simulink model "preliminary_Model"  (R2022b)
settings: Solver=FixedStepAuto  StartTime=0.0  StopTime=5  FixedStep=0.00001  RelTol=1e-3
model workspace (MAT data in the model file):
  g = 9.81
values from neighbouring files (symbols this model uses):
  A = [               0                ,        1        ,        0 ... (first row only)    [first_code.m]
  B = [ 0 ; -Km/(Ib+mw*l^2) ; Km*(Ib + Iw + mw*l^2)/(Iw*(Ib + mw*l^2)) ]    [first_code.m]
  C = [1 0 0; 0 1 0; 0 0 1]    [first_code.m]
  Cb = 1.02e-3    (= 0.00102)    [first_code.m]
  Cw = 0.05e-3    (= 5e-05)    [first_code.m]
  D = [0; 0; 0]    [first_code.m]
  Ib = 3.34e-3    (= 0.00334)    [first_code.m]
  Iw = 0.57e-3    (= 0.00057)    [first_code.m]
  l = 0.085    [first_code.m]
  lb = 0.075    [first_code.m]
  mb = 0.419    [first_code.m]
  mw = 0.204    [first_code.m]
libraries: slpidlib x3
settings Model: Creator=sAjaD  LastModifiedBy=Kian
settings SolverCC: AlgebraicLoopSolver=TrustRegion
settings DebuggingCC: UnconnectedInputMsg=warning  UnconnectedOutputMsg=warning  UnconnectedLineMsg=warning  SFMachineParentedDataDiag=warning  UnderSpecifiedDimensionMsg=warning
settings ModelReferenceCC: EnableRefExpFcnMdlSchedulingChecks=on

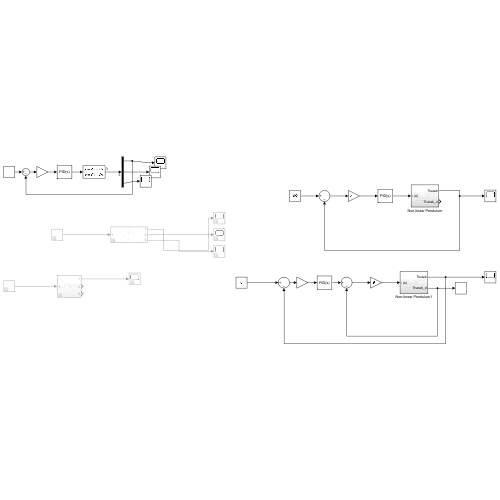
[thumbnail: Simulink's stored preview of the top-level diagram]
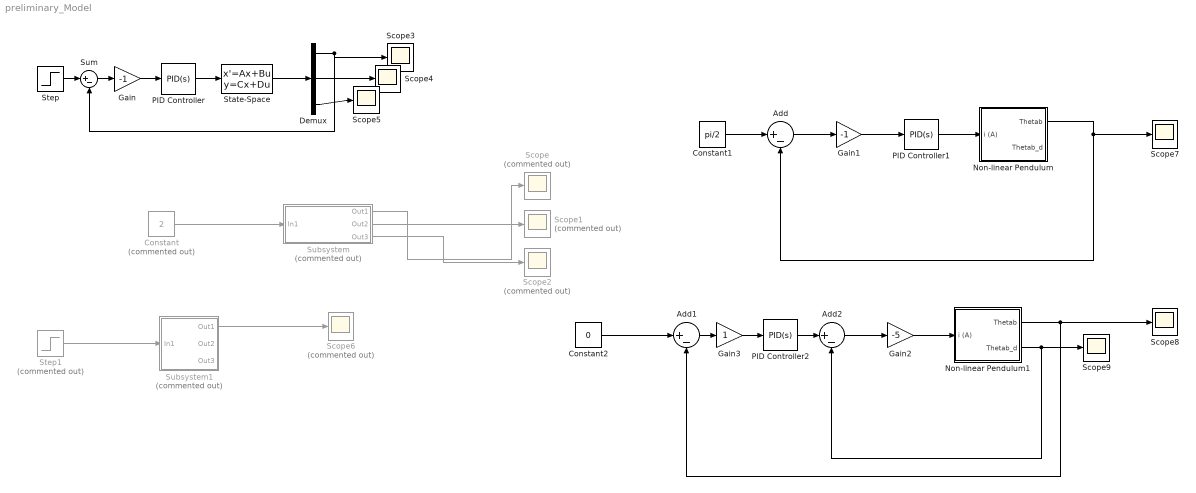
== system preliminary_Model ==
  Add : Sum  Inputs=|+-
  Add1 : Sum  Inputs=|+-
  Add2 : Sum  Inputs=|+-
  Constant : Constant  Commented=on  Value=2
  Constant1 : Constant  Value=pi/2
  Constant2 : Constant  Value=0
  Demux : Demux  Outputs=3
  Gain : Gain  Gain=-1
  Gain1 : Gain  Gain=-1
  Gain2 : Gain  Gain=-5
  Gain3 : Gain
  Non-linear Pendulum : Subsystem
  Non-linear Pendulum1 : Subsystem
  PID Controller : slpidlib/PID Controller  Controller=PID  Form=Parallel  TimeDomain=Continuous-time  UseExternalTs=off  SampleTime=-1  IntegratorMethod=Forward Euler  FilterMethod=Forward Euler  ControllerParametersSource=internal  P=100  I=0  UseKiTs=off  D=5  N=100  UseFilter=on  TunerSelectOption=Transfer Function Based (PID Tuner App)  InitialConditionSource=internal  InitialConditionForIntegrator=0  InitialConditionForFilter=0  DifferentiatorICPrevScaledInput=0  ExternalReset=none  TrackingMode=off  Kt=1  LimitOutput=off  SatLimitsSource=internal  UpperSaturationLimit=inf  LowerSaturationLimit=-inf  LinearizeAsGain=on  AntiWindupMode=none  Kb=1  LimitIntegrator=off  UpperIntegratorSaturationLimit=inf  LowerIntegratorSaturationLimit=-inf  POutMin=[]  POutMax=[]  IOutMin=[]  IOutMax=[]  DOutMin=[]  DOutMax=[]  NOutMin=[]  NOutMax=[]  SumOutMin=[]  SumOutMax=[]  SaturationOutMin=[]  SaturationOutMax=[]  PParamMin=[]  PParamMax=[]  IParamMin=[]  IParamMax=[]  DParamMin=[]  DParamMax=[]  NParamMin=[]  NParamMax=[]  KbParamMin=[]  KbParamMax=[]  KtParamMin=[]  KtParamMax=[]  KbOutMin=[]  KbOutMax=[]  KtOutMin=[]  KtOutMax=[]  IntegratorOutMin=[]  IntegratorOutMax=[]  FilterOutMin=[]  FilterOutMax=[]  SumI1OutMin=[]  SumI1OutMax=[]  SumI2OutMin=[]  SumI2OutMax=[]  SumI3OutMin=[]  SumI3OutMax=[]  SumI4OutMin=[]  SumI4OutMax=[]  SumDOutMin=[]  SumDOutMax=[]  DifferentiatorOutMin=[]  DifferentiatorOutMax=[]  FilterDiffOutCoefMin=[]  FilterDiffOutCoefMax=[]  ReciprocalOutMin=[]  ReciprocalOutMax=[]  SumDenOutMin=[]  SumDenOutMax=[]  SumNumOutMin=[]  SumNumOutMax=[]  DivideOutMin=[]  DivideOutMax=[]  UdiffTsProdOutMin=[]  UdiffTsProdOutMax=[]  NTsProdOutMin=[]  NTsProdOutMax=[]  UintegralTsProdOutMin=[]  UintegralTsProdOutMax=[]  UngainTsProdOutMin=[]  UngainTsProdOutMax=[]  ClampingZeroOutDataTypeStr=Inherit: Inherit via back propagation  ClampingZeroOutMin=[]  ClampingZeroOutMax=[]  FilterDenConstantOutDataTypeStr=Inherit: Inherit via back propagation  FilterDenConstantOutMin=[]  FilterDenConstantOutMax=[]  PCopyOutDataTypeStr=Inherit: Inherit via back propagation  PCopyOutMin=[]  PCopyOutMax=[]  NCopyOutDataTypeStr=Inherit: Inherit via back propagation  NCopyOutMin=[]  NCopyOutMax=[]  IntegratorContinuousStateAttributes=''  IntegratorStateMustResolveToSignalObject=off  IntegratorRTWStateStorageClass=Auto  FilterContinuousStateAttributes=''  FilterStateMustResolveToSignalObject=off  FilterRTWStateStorageClass=Auto  ParallelPVariant=InternalParameters  IdealPVariant=Disabled  IVariant=InternalParameters  DVariant=InternalParameters  IntegratorVariant=Continuous  SatVariant=Disabled  AWVariant=Passthrough  PCopyVariant=Disabled  TRVariant=Disabled  FdbkBlocksVariant=Forward  IdealPFdbkVariant=Disabled  SatFdbkVariant=Disabled  DerivativeFilterVariant=ContFilter  NVariant=InternalParameters  NCopyVariant=Disabled  FilterICVariant=InternalICsFilter  IntegratorICVariant=InternalICs  ExternalResetVariant=Disabled  TRSumVariant=Passthrough  SumFdbkVariant=Disabled  SumVariant=Sum_PID  TsampFilterVariant=InternalTs  TsampNgainVariant=Passthrough  TsampIntegralVariant=Passthrough  ExternalSaturationOutDataTypeStr=Inherit: Same as second input
  PID Controller1 : slpidlib/PID Controller  Controller=PID  Form=Parallel  TimeDomain=Continuous-time  UseExternalTs=off  SampleTime=-1  IntegratorMethod=Forward Euler  FilterMethod=Forward Euler  ControllerParametersSource=internal  P=100  I=0  UseKiTs=off  D=5  N=100  UseFilter=on  TunerSelectOption=Transfer Function Based (PID Tuner App)  InitialConditionSource=internal  InitialConditionForIntegrator=0  InitialConditionForFilter=0  DifferentiatorICPrevScaledInput=0  ExternalReset=none  TrackingMode=off  Kt=1  LimitOutput=off  SatLimitsSource=internal  UpperSaturationLimit=inf  LowerSaturationLimit=-inf  LinearizeAsGain=on  AntiWindupMode=none  Kb=1  LimitIntegrator=off  UpperIntegratorSaturationLimit=inf  LowerIntegratorSaturationLimit=-inf  POutMin=[]  POutMax=[]  IOutMin=[]  IOutMax=[]  DOutMin=[]  DOutMax=[]  NOutMin=[]  NOutMax=[]  SumOutMin=[]  SumOutMax=[]  SaturationOutMin=[]  SaturationOutMax=[]  PParamMin=[]  PParamMax=[]  IParamMin=[]  IParamMax=[]  DParamMin=[]  DParamMax=[]  NParamMin=[]  NParamMax=[]  KbParamMin=[]  KbParamMax=[]  KtParamMin=[]  KtParamMax=[]  KbOutMin=[]  KbOutMax=[]  KtOutMin=[]  KtOutMax=[]  IntegratorOutMin=[]  IntegratorOutMax=[]  FilterOutMin=[]  FilterOutMax=[]  SumI1OutMin=[]  SumI1OutMax=[]  SumI2OutMin=[]  SumI2OutMax=[]  SumI3OutMin=[]  SumI3OutMax=[]  SumI4OutMin=[]  SumI4OutMax=[]  SumDOutMin=[]  SumDOutMax=[]  DifferentiatorOutMin=[]  DifferentiatorOutMax=[]  FilterDiffOutCoefMin=[]  FilterDiffOutCoefMax=[]  ReciprocalOutMin=[]  ReciprocalOutMax=[]  SumDenOutMin=[]  SumDenOutMax=[]  SumNumOutMin=[]  SumNumOutMax=[]  DivideOutMin=[]  DivideOutMax=[]  UdiffTsProdOutMin=[]  UdiffTsProdOutMax=[]  NTsProdOutMin=[]  NTsProdOutMax=[]  UintegralTsProdOutMin=[]  UintegralTsProdOutMax=[]  UngainTsProdOutMin=[]  UngainTsProdOutMax=[]  ClampingZeroOutDataTypeStr=Inherit: Inherit via back propagation  ClampingZeroOutMin=[]  ClampingZeroOutMax=[]  FilterDenConstantOutDataTypeStr=Inherit: Inherit via back propagation  FilterDenConstantOutMin=[]  FilterDenConstantOutMax=[]  PCopyOutDataTypeStr=Inherit: Inherit via back propagation  PCopyOutMin=[]  PCopyOutMax=[]  NCopyOutDataTypeStr=Inherit: Inherit via back propagation  NCopyOutMin=[]  NCopyOutMax=[]  IntegratorContinuousStateAttributes=''  IntegratorStateMustResolveToSignalObject=off  IntegratorRTWStateStorageClass=Auto  FilterContinuousStateAttributes=''  FilterStateMustResolveToSignalObject=off  FilterRTWStateStorageClass=Auto  ParallelPVariant=InternalParameters  IdealPVariant=Disabled  IVariant=InternalParameters  DVariant=InternalParameters  IntegratorVariant=Continuous  SatVariant=Disabled  AWVariant=Passthrough  PCopyVariant=Disabled  TRVariant=Disabled  FdbkBlocksVariant=Forward  IdealPFdbkVariant=Disabled  SatFdbkVariant=Disabled  DerivativeFilterVariant=ContFilter  NVariant=InternalParameters  NCopyVariant=Disabled  FilterICVariant=InternalICsFilter  IntegratorICVariant=InternalICs  ExternalResetVariant=Disabled  TRSumVariant=Passthrough  SumFdbkVariant=Disabled  SumVariant=Sum_PID  TsampFilterVariant=InternalTs  TsampNgainVariant=Passthrough  TsampIntegralVariant=Passthrough  ExternalSaturationOutDataTypeStr=Inherit: Same as second input
  PID Controller2 : slpidlib/PID Controller  Controller=PID  Form=Parallel  TimeDomain=Continuous-time  UseExternalTs=off  SampleTime=-1  IntegratorMethod=Forward Euler  FilterMethod=Forward Euler  ControllerParametersSource=internal  P=21  I=59  UseKiTs=off  D=0.66  N=1925  UseFilter=on  TunerSelectOption=Transfer Function Based (PID Tuner App)  InitialConditionSource=internal  InitialConditionForIntegrator=0  InitialConditionForFilter=0  DifferentiatorICPrevScaledInput=0  ExternalReset=none  TrackingMode=off  Kt=1  LimitOutput=off  SatLimitsSource=internal  UpperSaturationLimit=inf  LowerSaturationLimit=-inf  LinearizeAsGain=on  AntiWindupMode=none  Kb=1  LimitIntegrator=off  UpperIntegratorSaturationLimit=inf  LowerIntegratorSaturationLimit=-inf  POutMin=[]  POutMax=[]  IOutMin=[]  IOutMax=[]  DOutMin=[]  DOutMax=[]  NOutMin=[]  NOutMax=[]  SumOutMin=[]  SumOutMax=[]  SaturationOutMin=[]  SaturationOutMax=[]  PParamMin=[]  PParamMax=[]  IParamMin=[]  IParamMax=[]  DParamMin=[]  DParamMax=[]  NParamMin=[]  NParamMax=[]  KbParamMin=[]  KbParamMax=[]  KtParamMin=[]  KtParamMax=[]  KbOutMin=[]  KbOutMax=[]  KtOutMin=[]  KtOutMax=[]  IntegratorOutMin=[]  IntegratorOutMax=[]  FilterOutMin=[]  FilterOutMax=[]  SumI1OutMin=[]  SumI1OutMax=[]  SumI2OutMin=[]  SumI2OutMax=[]  SumI3OutMin=[]  SumI3OutMax=[]  SumI4OutMin=[]  SumI4OutMax=[]  SumDOutMin=[]  SumDOutMax=[]  DifferentiatorOutMin=[]  DifferentiatorOutMax=[]  FilterDiffOutCoefMin=[]  FilterDiffOutCoefMax=[]  ReciprocalOutMin=[]  ReciprocalOutMax=[]  SumDenOutMin=[]  SumDenOutMax=[]  SumNumOutMin=[]  SumNumOutMax=[]  DivideOutMin=[]  DivideOutMax=[]  UdiffTsProdOutMin=[]  UdiffTsProdOutMax=[]  NTsProdOutMin=[]  NTsProdOutMax=[]  UintegralTsProdOutMin=[]  UintegralTsProdOutMax=[]  UngainTsProdOutMin=[]  UngainTsProdOutMax=[]  ClampingZeroOutDataTypeStr=Inherit: Inherit via back propagation  ClampingZeroOutMin=[]  ClampingZeroOutMax=[]  FilterDenConstantOutDataTypeStr=Inherit: Inherit via back propagation  FilterDenConstantOutMin=[]  FilterDenConstantOutMax=[]  PCopyOutDataTypeStr=Inherit: Inherit via back propagation  PCopyOutMin=[]  PCopyOutMax=[]  NCopyOutDataTypeStr=Inherit: Inherit via back propagation  NCopyOutMin=[]  NCopyOutMax=[]  IntegratorContinuousStateAttributes=''  IntegratorStateMustResolveToSignalObject=off  IntegratorRTWStateStorageClass=Auto  FilterContinuousStateAttributes=''  FilterStateMustResolveToSignalObject=off  FilterRTWStateStorageClass=Auto  ParallelPVariant=InternalParameters  IdealPVariant=Disabled  IVariant=InternalParameters  DVariant=InternalParameters  IntegratorVariant=Continuous  SatVariant=Disabled  AWVariant=Passthrough  PCopyVariant=Disabled  TRVariant=Disabled  FdbkBlocksVariant=Forward  IdealPFdbkVariant=Disabled  SatFdbkVariant=Disabled  DerivativeFilterVariant=ContFilter  NVariant=InternalParameters  NCopyVariant=Disabled  FilterICVariant=InternalICsFilter  IntegratorICVariant=InternalICs  ExternalResetVariant=Disabled  TRSumVariant=Passthrough  SumFdbkVariant=Disabled  SumVariant=Sum_PID  TsampFilterVariant=InternalTs  TsampNgainVariant=Passthrough  TsampIntegralVariant=Passthrough  ExternalSaturationOutDataTypeStr=Inherit: Same as second input
  Scope{,1..2,6} (4 alike) : Scope  Commented=on
  Scope{3..5,7..9} (6 alike) : Scope
  State-Space : StateSpace  A=A  B=B  C=C  D=D  InitialCondition=[pi ; 0 ; 0]
  Step : Step  After=0  SampleTime=0
  Step1 : Step  Commented=on  After=10  SampleTime=0
  Subsystem : Subsystem  Commented=on  InitFcn=|
      | mb = 0.419 ; %% kg : pendulum body  
      | mw = 0.204 ; %% kg : wheel masses
      | l = 0.085 ; %% m : Distance between the motor axis and the pivot point
      | lb = 0.075 ; %% m  : Distance between the center of amss of the pendulum body and the pivot point 
      | Ib = 3.34e-3 ; %% kg.m2 : Moment of inertia of the pendulum body 
      | Iw = 0.57e-3 ; %% kg.m2 : Moment of inertia of the wheel and the motor rotor around the rotational axis of the motor
      | Cb = 1.02e-3 ; %% kg.m2.s-1 : Dynamic friction coefficient of the wheel 
      | Cw = 0.05e-3 ; %% kg.m2.s-1 : Dynamic friction coefficient of the pendulum body 
      | % %%Tm ; %% N.m : Torque pruduced by the Motor
      | Km = 25.1e-3 ; %% N.m.A-1 : Torque constant of the brushless DC motor 
      | % %%u  ; %% A : Current input
      | g = 9.81 ; %% m.s-2 : Gravitational Constant
      | dh = 0.5 ; %% N.m : Disturbant Torque
      settings: OpenFcn=|
      | mb = 0.419 ; %% kg : pendulum body
      | mw = 0.204 ; %% kg : wheel masses
      | l = 0.085 ; %% m : Distance between the motor axis and the pivot point
      | lb = 0.075 ; %% m  : Distance between the center of amss of the pendulum body and the pivot point
      | Ib = 3.34e-3 ; %% kg.m2 : Moment of inertia of the pendulum body
      | Iw = 0.57e-3 ; %% kg.m2 : Moment of inertia of the wheel and the motor rotor around the rotational axis of the motor
      | Cb = 1.02e-3 ; %% kg.m2.s-1 : Dynamic friction coefficient of the wheel
      | Cw = 0.05e-3 ; %% kg.m2.s-1 : Dynamic friction coefficient of the pendulum body
      | % %%Tm ; %% N.m : Torque pruduced by the Motor
      | Km = 25.1e-3 ; %% N.m.A-1 : Torque constant of the brushless DC motor
      | % %%u  ; %% A : Current input
      | g = 9.81 ; %% m.s-2 : Gravitational Constant
      | dh = 0.5 ; %% N.m : Disturbant Torque
  Subsystem1 : Subsystem  Commented=on
  Sum : Sum  Inputs=|+-
  wires:
  Constant/1 -> Subsystem/1(In1)
  Subsystem/1(Out1) -> Scope/1
  Subsystem/2(Out2) -> Scope1/1
  Subsystem/3(Out3) -> Scope2/1
  State-Space/1 -> Demux/1
  Demux/3 -> Scope5/1
  Demux/2 -> Scope4/1
  Demux/1 -> Scope3/1, Sum/2
  Step/1 -> Sum/1
  Sum/1 -> Gain/1
  PID Controller/1 -> State-Space/1
  Gain/1 -> PID Controller/1
  Step1/1 -> Subsystem1/1(In1)
  Subsystem1/1(Out1) -> Scope6/1
  Constant1/1 -> Add/1
  Add/1 -> Gain1/1
  Gain1/1 -> PID Controller1/1
  Non-linear Pendulum/1(Thetab) -> Add/2, Scope7/1
  PID Controller1/1 -> Non-linear Pendulum/1(i (A))
  Gain2/1 -> Non-linear Pendulum1/1(i (A))
  Non-linear Pendulum1/1(Thetab) -> Scope8/1, Add1/2
  Add1/1 -> Gain3/1
  Constant2/1 -> Add1/1
  Non-linear Pendulum1/2(Thetab_d) -> Add2/2, Scope9/1
  Add2/1 -> Gain2/1
  PID Controller2/1 -> Add2/1
  Gain3/1 -> PID Controller2/1

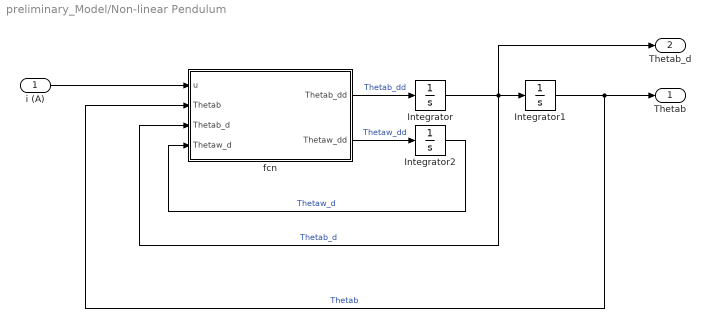
== system preliminary_Model/Non-linear Pendulum ==
  i (A) : Inport
  Integrator : Integrator
  Integrator1 : Integrator  InitialCondition=pi
  Integrator2 : Integrator
  fcn : MATLAB Function  TreatAsAtomicUnit=on
  Thetab : Outport
  Thetab_d : Outport  Port=2
  wires:
  Integrator/1 -> Thetab_d/1, Integrator1/1, fcn/3(Thetab_d)  "Thetab_d"
  fcn/2(Thetaw_dd) -> Integrator2/1  "Thetaw_dd"
  Integrator1/1 -> Thetab/1, fcn/2(Thetab)  "Thetab"
  Integrator2/1 -> fcn/4(Thetaw_d)  "Thetaw_d"
  fcn/1(Thetab_dd) -> Integrator/1  "Thetab_dd"
  i (A)/1 -> fcn/1(u)

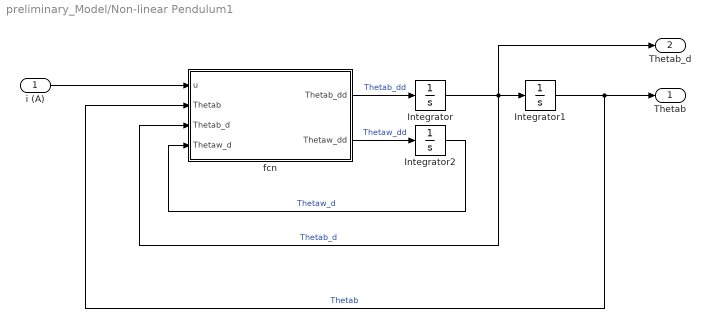
== system preliminary_Model/Non-linear Pendulum1 ==
  i (A) : Inport
  Integrator : Integrator  InitialCondition=pi/3
  Integrator1 : Integrator
  Integrator2 : Integrator
  fcn : MATLAB Function  TreatAsAtomicUnit=on
  Thetab : Outport
  Thetab_d : Outport  Port=2
  wires:
  i (A)/1 -> fcn/1(u)
  fcn/1(Thetab_dd) -> Integrator/1  "Thetab_dd"
  Integrator2/1 -> fcn/4(Thetaw_d)  "Thetaw_d"
  Integrator1/1 -> fcn/2(Thetab), Thetab/1  "Thetab"
  fcn/2(Thetaw_dd) -> Integrator2/1  "Thetaw_dd"
  Integrator/1 -> fcn/3(Thetab_d), Integrator1/1, Thetab_d/1  "Thetab_d"

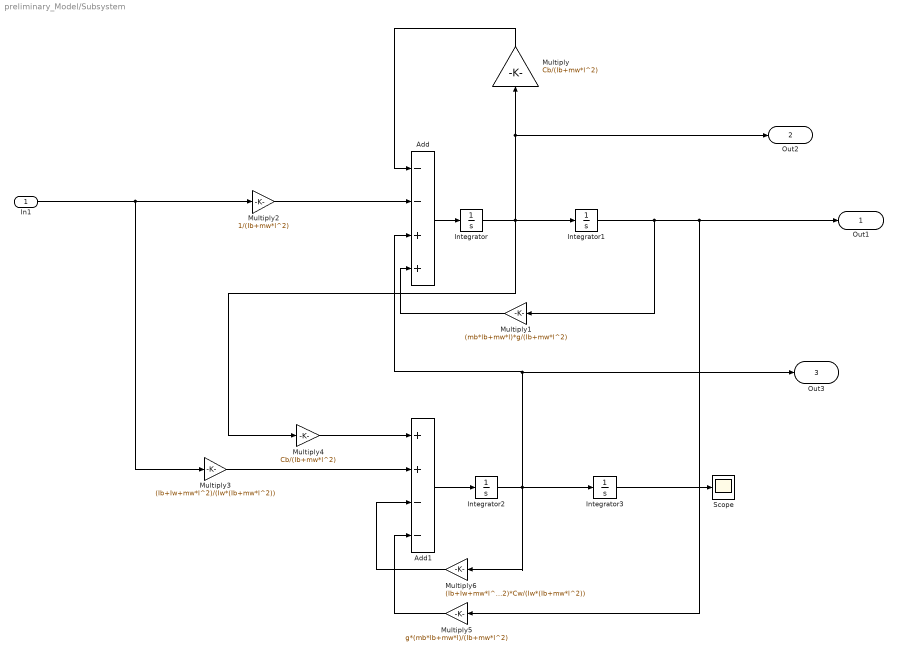
== system preliminary_Model/Subsystem ==
  In1 : Inport
  Add : Sum  Inputs=--++
  Add1 : Sum  Inputs=++--
  Integrator : Integrator
  Integrator1 : Integrator  InitialCondition=45
  Integrator2 : Integrator
  Integrator3 : Integrator
  Multiply : Gain  Gain=Cb/(Ib+mw*l^2)
  Multiply1 : Gain  Gain=(mb*lb+mw*l)*g/(Ib+mw*l^2)
  Multiply2 : Gain  Gain=1/(Ib+mw*l^2)
  Multiply3 : Gain  Gain=(Ib+Iw+mw*l^2)/(Iw*(Ib+mw*l^2))
  Multiply4 : Gain  Gain=Cb/(Ib+mw*l^2)
  Multiply5 : Gain  Gain=g*(mb*lb+mw*l)/(Ib+mw*l^2)
  Multiply6 : Gain  Gain=(Ib+Iw+mw*l^2)*Cw/(Iw*(Ib+mw*l^2))
  Scope : Scope
  Out1 : Outport
  Out2 : Outport  Port=2
  Out3 : Outport  Port=3
  wires:
  Integrator1/1 -> Multiply1/1, Multiply5/1, Out1/1
  Integrator/1 -> Multiply4/1, Out2/1, Multiply/1, Integrator1/1
  Integrator2/1 -> Multiply6/1, Add/3, Out3/1, Integrator3/1
  Add/1 -> Integrator/1
  Multiply/1 -> Add/1
  Multiply1/1 -> Add/4
  Multiply2/1 -> Add/2
  Add1/1 -> Integrator2/1
  In1/1 -> Multiply3/1, Multiply2/1
  Multiply3/1 -> Add1/2
  Multiply4/1 -> Add1/1
  Multiply6/1 -> Add1/3
  Multiply5/1 -> Add1/4
  Integrator3/1 -> Scope/1

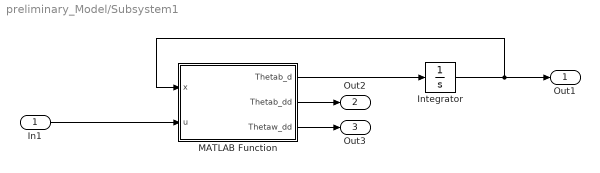
== system preliminary_Model/Subsystem1 ==
  In1 : Inport
  Integrator : Integrator
  MATLAB Function : MATLAB Function  TreatAsAtomicUnit=on
  Out1 : Outport
  Out2 : Outport  Port=2
  Out3 : Outport  Port=3
  wires:
  Integrator/1 -> Out1/1, MATLAB Function/1(x)
  MATLAB Function/1(Thetab_d) -> Integrator/1
  In1/1 -> MATLAB Function/2(u)
  MATLAB Function/3(Thetaw_dd) -> Out3/1
  MATLAB Function/2(Thetab_dd) -> Out2/1

== matlab function preliminary_Model/Non-linear Pendulum/fcn ==
  data: u input; Thetab input; Thetab_d input; Thetaw_d input; Thetab_dd output; Thetaw_dd output
function [Thetab_dd , Thetaw_dd] = fcn(u , Thetab , Thetab_d , Thetaw_d)

mb = 0.419 ; %% kg : pendulum body
mw = 0.204 ; %% kg : wheel masses
l = 0.085 ; %% m : Distance between the motor axis and the pivot point
lb = 0.075 ; %% m  : Distance between the center of amss of the pendulum body and the pivot point
Ib = 3.34e-3 ; %% kg.m2 : Moment of inertia of the pendulum body
Iw = 0.57e-3 ; %% kg.m2 : Moment of inertia of the wheel and the motor rotor around the rotational axis of the motor
Cb = 1.02e-3 ; %% kg.m2.s-1 : Dynamic friction coefficient of the wheel
Cw = 0.05e-3 ; %% kg.m2.s-1 : Dynamic friction coefficient of the pendulum body
%%Tm ; %% N.m : Torque pruduced by the Motor
Km = 25.1e-3 ; %% N.m.A-1 : Torque constant of the brushless DC motor
%%u  ; %% A : Current input
g = 9.81 ; %% m.s-2 : Gravitational Constant

Thetab_dd = ((mb*lb + mw*l)*g*sin(Thetab) - Km*u - Cb*Thetab_d + Cw*Thetaw_d ) / (Ib + mw*l^2) ;

Thetaw_dd = ( (Ib + Iw + mw*l^2)*(Km*u - Cw*Thetaw_d))/(Iw *(Ib + mw*l^2))...
    - ((mb*lb + mw*l)*g*sin(Thetab) - Cb*Thetab_d)/(Ib + mw*l^2) ;
end

== matlab function preliminary_Model/Subsystem1/MATLAB Function ==
  data: x input; u input; Thetab_d output; Thetab_dd output; Thetaw_dd output
function [Thetab_d,  Thetab_dd,  Thetaw_dd] = fcn(x,u)
    Thetab_d = x(2,1) ; 
    Thetab_dd = ((mb*lb + mw*l)*g*sin(x(1,1)) - Km*u - Cb*x(2,1) + Cw*x(3,1) ) / (Ib + mw*l^2) ; 
    Thetaw_dd = ( (Ib+Iw+mw*l^2)*(Km*u - Cw*x(3,1)))/(Iw*(Ib+mw*l^2)) - ( (mb*lb + mw*l)*g*sin(x(1))-Cb*x(2,1))/(Ib + mw*l^2) ;

== matlab function preliminary_Model/Non-linear Pendulum1/fcn ==
  data: u input; Thetab input; Thetab_d input; Thetaw_d input; Thetab_dd output; Thetaw_dd output
function [Thetab_dd , Thetaw_dd] = fcn(u , Thetab , Thetab_d , Thetaw_d)

mb = 0.419 ; %% kg : pendulum body
mw = 0.204 ; %% kg : wheel masses
l = 0.085 ; %% m : Distance between the motor axis and the pivot point
lb = 0.075 ; %% m  : Distance between the center of amss of the pendulum body and the pivot point
Ib = 3.34e-3 ; %% kg.m2 : Moment of inertia of the pendulum body
Iw = 0.57e-3 ; %% kg.m2 : Moment of inertia of the wheel and the motor rotor around the rotational axis of the motor
Cb = 1.02e-3 ; %% kg.m2.s-1 : Dynamic friction coefficient of the wheel
Cw = 0.05e-3 ; %% kg.m2.s-1 : Dynamic friction coefficient of the pendulum body
%%Tm ; %% N.m : Torque pruduced by the Motor
Km = 25.1e-3 ; %% N.m.A-1 : Torque constant of the brushless DC motor
%%u  ; %% A : Current input
g = 9.81 ; %% m.s-2 : Gravitational Constant

Thetab_dd = ((mb*lb + mw*l)*g*sin(Thetab) - Km*u - Cb*Thetab_d + Cw*Thetaw_d ) / (Ib + mw*l^2) ;

Thetaw_dd = ( (Ib + Iw + mw*l^2)*(Km*u - Cw*Thetaw_d))/(Iw *(Ib + mw*l^2))...
    - ((mb*lb + mw*l)*g*sin(Thetab) - Cb*Thetab_d)/(Ib + mw*l^2) ;
end
